simulink model "c_station_v2"  (R2019a)
settings: Solver=VariableStepAuto  StartTime=0.0  StopTime=604800  MaxStep=3600  RelTol=1e-3  AbsTol=1e-3  EnableMultiTasking=on
values from neighbouring files (symbols this model uses):
  conf = gasConfig()    [gas_v1.m]
  loadControlFlag = "on"    [gas_v1.m]
  valveControlFlag = "on"    [gas_v1.m]
undefined symbols (not defined in the file or in its folder): f, lineParm, loadParm, valveParm
libraries: fl_lib x31, gasLibrary x13, nesl_utility x13, instrumentlib x6, SimscapeFluids_lib x1
(part 1 of 3)
settings Model: Creator=dzimm  LastModifiedBy=brandt
settings SolverCC: AutoScaleAbsTol=off
settings DataIOCC: LimitDataPoints=on  MaxDataPoints=10000  ReturnWorkspaceOutputs=off
settings OptimizationCC: LifeSpan=inf
settings DebuggingCC: AllowSymbolicDim=off  PregeneratedLibrarySubsystemCodeDiagnostic=none  SFUnexpectedBacktrackingDiag=warning  SFNoUnconditionalDefaultTransitionDiag=warning  SFExecutionAtInitializationDiag=none  ArithmeticOperatorsInVariantConditions=warning
settings SFSimCC: SimUseLocalCustomCode=off
settings RTWCC: RTWUseLocalCustomCode=off
settings CodeAppCC: StateflowObjectComments=on
settings GRTTargetCC: TargetLangStandard=C89/C90 (ANSI)  GeneratePreprocessorConditionals=Disable all
settings ConfigComp: CovMetricSettings=dw  CovHtmlReporting=on  CovSaveCumulativeToWorkspaceVar=on  CovSaveSingleToWorkspaceVar=on  CovExternalEMLEnable=off  CovSFcnEnable=off
settings SimscapeCC: SimscapeLogType=all  SimscapeLogOpenViewer=on  SimscapeLogLimitData=off  SimscapeLogDataHistory=10000  SimscapeUseOperatingPoints=on  SimscapeOperatingPoint=op

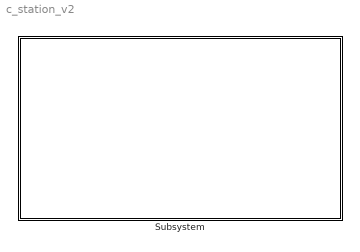
== system c_station_v2 ==
  Subsystem : Subsystem
